simulink subsystem "brakeregen"  (R2022b)
settings: Solver=VariableStepAuto  StartTime=0.0  StopTime=10.0  RelTol=1e-3
settings Model: Creator=serga  LastModifiedBy=serga

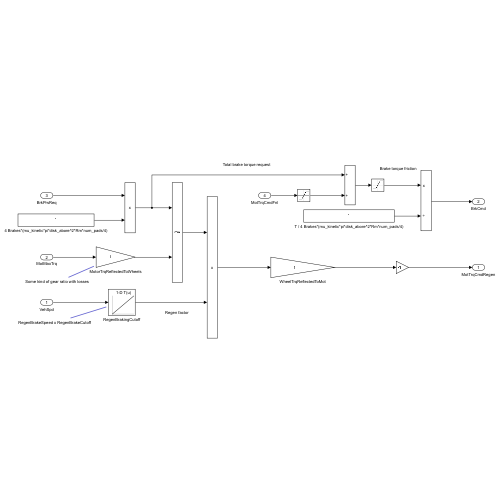
[thumbnail: Simulink's stored preview of the top-level diagram]
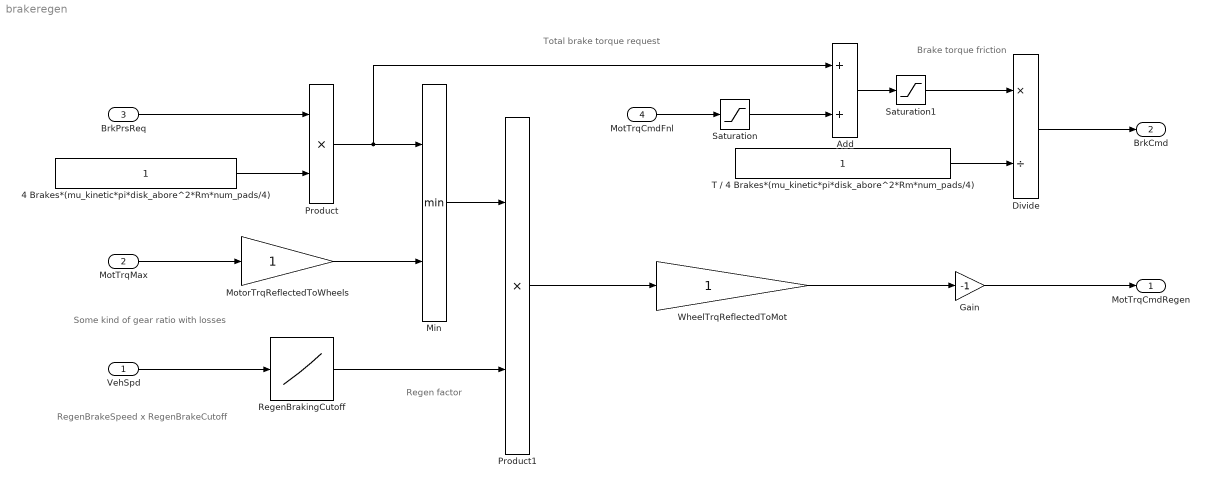
== system brakeregen ==
  note: Regen factor
  note: Total brake torque request
  note: Brake torque friction
  note: Some kind of gear ratio with losses
  note: RegenBrakeSpeed x RegenBrakeCutoff
  VehSpd : Inport
  MotTrqMax : Inport  Port=2
  BrkPrsReq : Inport  Port=3
  MotTrqCmdFnl : Inport  Port=4
  4 Brakes*(mu_kinetic*pi*disk_abore^2*Rm*num_pads/4) : Constant
  Add : Sum
  Divide : Product  Inputs=*/
  Gain : Gain  Gain=-1
  Min : MinMax  Inputs=2
  MotorTrqReflectedToWheels : Gain
  Product : Product
  Product1 : Product
  RegenBrakingCutoff : Lookup_n-D  NumberOfTableDimensions=1  BreakpointsForDimension1=[5 9]  Table=[0 1]  InternalRulePriority=Speed  RndMeth=Simplest
  Saturation : Saturate  LowerLimit=-inf
  Saturation1 : Saturate  UpperLimit=inf  LowerLimit=0
  T / 4 Brakes*(mu_kinetic*pi*disk_abore^2*Rm*num_pads/4) : Constant
  WheelTrqReflectedToMot : Gain
  MotTrqCmdRegen : Outport
  BrkCmd : Outport  Port=2
  wires:
  BrkPrsReq/1 -> Product/1
  4 Brakes*(mu_kinetic*pi*disk_abore^2*Rm*num_pads/4)/1 -> Product/2
  MotTrqMax/1 -> MotorTrqReflectedToWheels/1
  VehSpd/1 -> RegenBrakingCutoff/1
  MotorTrqReflectedToWheels/1 -> Min/2
  Product/1 -> Add/1, Min/1
  RegenBrakingCutoff/1 -> Product1/2
  Min/1 -> Product1/1
  MotTrqCmdFnl/1 -> Saturation/1
  Saturation/1 -> Add/2
  Product1/1 -> WheelTrqReflectedToMot/1
  WheelTrqReflectedToMot/1 -> Gain/1
  Add/1 -> Saturation1/1
  Saturation1/1 -> Divide/1
  Divide/1 -> BrkCmd/1
  T / 4 Brakes*(mu_kinetic*pi*disk_abore^2*Rm*num_pads/4)/1 -> Divide/2
  Gain/1 -> MotTrqCmdRegen/1
